simulink model "dft_polyphase_8_channel_builtin_blocks"  (R2018b)
settings: Solver=FixedStepDiscrete  StartTime=0.0  StopTime=t(end)  RelTol=1e-3  EnableMultiTasking=on
InitFcn:
  | M = 8; % Number of channels in the filter bank.
  | N = 8;  % Number of taps in each FIR filter.
  | n_out = 4000; % Number of output samples
  | datatypeselector = 'hdl'; % 'double' 'single' 'hdl' 'dsp'
  | [T,B,U,b,u,t,fs] = generate_inputs(M,N,n_out,datatypeselector);
values from neighbouring files (symbols this model uses):
  B = cast(B,'like',T.fir_filter.coeff)    [generate_inputs.m]
  fs = n    [generate_inputs.m]
libraries: dft_polyphase_channelizer_library x8, dspsrcs4 x1, dspxfrm3 x1
settings Model: Creator=tbryan  LastModifiedBy=tbryan
settings SolverCC: AutoInsertRateTranBlk=on
settings OptimizationCC: LifeSpan=inf
settings DebuggingCC: AllowSymbolicDim=off  SFUnexpectedBacktrackingDiag=warning  SFNoUnconditionalDefaultTransitionDiag=warning  SFExecutionAtInitializationDiag=none
settings SFSimCC: SimUseLocalCustomCode=off
settings RTWCC: RTWUseLocalCustomCode=off
settings CodeAppCC: StateflowObjectComments=on
settings GRTTargetCC: TargetLangStandard=C89/C90 (ANSI)  GeneratePreprocessorConditionals=Disable all
settings ConfigComp: CovMetricSettings=dw  CovHtmlReporting=on  CovSaveCumulativeToWorkspaceVar=on  CovSaveSingleToWorkspaceVar=on  CovExternalEMLEnable=off

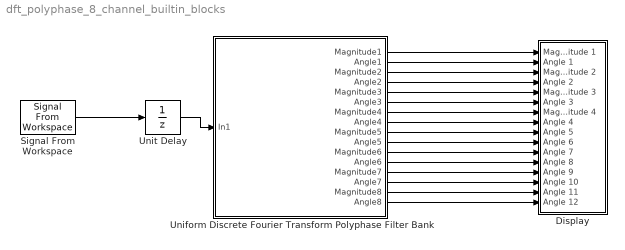
== system dft_polyphase_8_channel_builtin_blocks ==
  Display : Subsystem
  Signal From Workspace : dspsrcs4/Signal From Workspace  X=u  Ts=1/fs  nsamps=1  OutputAfterFinalValue=Setting to zero  ignoreOrWarnInputAndFrameLengths=off  OutputFrames=off
  Uniform Discrete Fourier Transform Polyphase Filter Bank : Subsystem
  Unit Delay : UnitDelay  SampleTime=-1
  wires:
  Signal From Workspace/1 -> Unit Delay/1
  Unit Delay/1 -> Uniform Discrete Fourier Transform Polyphase Filter Bank/1(In1)
  Uniform Discrete Fourier Transform Polyphase Filter Bank/1(Magnitude1) -> Display/1(Magnitude 1)
  Uniform Discrete Fourier Transform Polyphase Filter Bank/2(Angle1) -> Display/2(Angle 1)
  Uniform Discrete Fourier Transform Polyphase Filter Bank/3(Magnitude2) -> Display/3(Magnitude 2)
  Uniform Discrete Fourier Transform Polyphase Filter Bank/4(Angle2) -> Display/4(Angle 2)
  Uniform Discrete Fourier Transform Polyphase Filter Bank/5(Magnitude3) -> Display/5(Magnitude 3)
  Uniform Discrete Fourier Transform Polyphase Filter Bank/6(Angle3) -> Display/6(Angle 3)
  Uniform Discrete Fourier Transform Polyphase Filter Bank/7(Magnitude4) -> Display/7(Magnitude 4)
  Uniform Discrete Fourier Transform Polyphase Filter Bank/8(Angle4) -> Display/8(Angle 4)
  Uniform Discrete Fourier Transform Polyphase Filter Bank/9(Magnitude5) -> Display/9(Angle 5)
  Uniform Discrete Fourier Transform Polyphase Filter Bank/10(Angle5) -> Display/10(Angle 6)
  Uniform Discrete Fourier Transform Polyphase Filter Bank/11(Magnitude6) -> Display/11(Angle 7)
  Uniform Discrete Fourier Transform Polyphase Filter Bank/12(Angle6) -> Display/12(Angle 8)
  Uniform Discrete Fourier Transform Polyphase Filter Bank/13(Magnitude7) -> Display/13(Angle 9)
  Uniform Discrete Fourier Transform Polyphase Filter Bank/14(Angle7) -> Display/14(Angle 10)
  Uniform Discrete Fourier Transform Polyphase Filter Bank/15(Magnitude8) -> Display/15(Angle 11)
  Uniform Discrete Fourier Transform Polyphase Filter Bank/16(Angle8) -> Display/16(Angle 12)

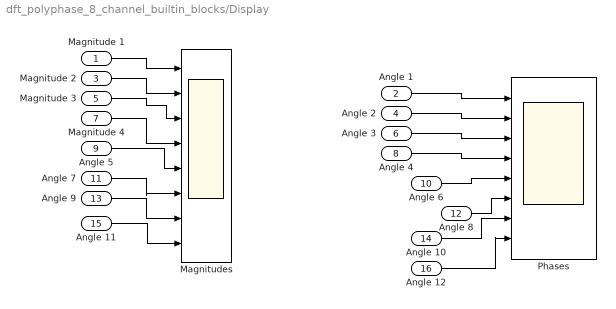
== system dft_polyphase_8_channel_builtin_blocks/Display ==
  Magnitude 1 : Inport
  Angle 1 : Inport  Port=2
  Magnitude 2 : Inport  Port=3
  Angle 2 : Inport  Port=4
  Magnitude 3 : Inport  Port=5
  Angle 3 : Inport  Port=6
  Magnitude 4 : Inport  Port=7
  Angle 4 : Inport  Port=8
  Angle 5 : Inport  Port=9
  Angle 6 : Inport  Port=10
  Angle 7 : Inport  Port=11
  Angle 8 : Inport  Port=12
  Angle 9 : Inport  Port=13
  Angle 10 : Inport  Port=14
  Angle 11 : Inport  Port=15
  Angle 12 : Inport  Port=16
  Magnitudes : Scope  NumInputPorts=8
  Phases : Scope  NumInputPorts=8
  wires:
  Angle 3/1 -> Phases/3
  Magnitude 2/1 -> Magnitudes/2
  Magnitude 1/1 -> Magnitudes/1
  Magnitude 4/1 -> Magnitudes/4
  Angle 2/1 -> Phases/2
  Angle 4/1 -> Phases/4
  Magnitude 3/1 -> Magnitudes/3
  Angle 1/1 -> Phases/1
  Angle 5/1 -> Magnitudes/5
  Angle 7/1 -> Magnitudes/6
  Angle 9/1 -> Magnitudes/7
  Angle 11/1 -> Magnitudes/8
  Angle 6/1 -> Phases/5
  Angle 8/1 -> Phases/6
  Angle 10/1 -> Phases/7
  Angle 12/1 -> Phases/8

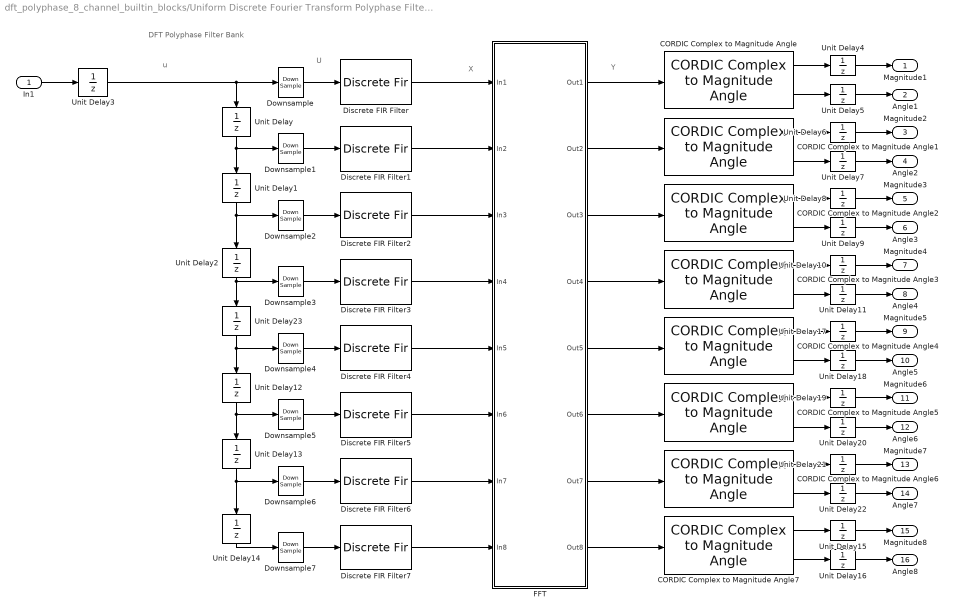
== system dft_polyphase_8_channel_builtin_blocks/Uniform Discrete Fourier Transform Polyphase Filter Bank ==
  note: DFT Polyphase Filter Bank
  note: U
  note: u
  note: X
  note: Y
  In1 : Inport
   CORDIC Complex to Magnitude Angle{,1..7} (8 alike) : dft_polyphase_channelizer_library/CORDIC Complex to Magnitude Angle  SystemSampleTime=-1
  Discrete FIR Filter : DiscreteFir  Coefficients=B(1,:)  AccumDataTypeStr=Inherit: Same as product output
  Discrete FIR Filter1 : DiscreteFir  Coefficients=B(2,:)  AccumDataTypeStr=Inherit: Same as product output
  Discrete FIR Filter2 : DiscreteFir  Coefficients=B(3,:)  AccumDataTypeStr=Inherit: Same as product output
  Discrete FIR Filter3 : DiscreteFir  Coefficients=B(4,:)  AccumDataTypeStr=Inherit: Same as product output
  Discrete FIR Filter4 : DiscreteFir  Coefficients=B(5,:)  AccumDataTypeStr=Inherit: Same as product output
  Discrete FIR Filter5 : DiscreteFir  Coefficients=B(6,:)  AccumDataTypeStr=Inherit: Same as product output
  Discrete FIR Filter6 : DiscreteFir  Coefficients=B(7,:)  AccumDataTypeStr=Inherit: Same as product output
  Discrete FIR Filter7 : DiscreteFir  Coefficients=B(8,:)  AccumDataTypeStr=Inherit: Same as product output
  Downsample{,1..7} (8 alike) : DownSample  N=M  RateOptions=Allow multirate processing
  FFT : Subsystem
      mask Display: disp('IDFT')
  Unit Delay{,1..23} (24 alike) : UnitDelay  SampleTime=-1
  Magnitude1 : Outport
  Angle1 : Outport  Port=2
  Magnitude2 : Outport  Port=3
  Angle2 : Outport  Port=4
  Magnitude3 : Outport  Port=5
  Angle3 : Outport  Port=6
  Magnitude4 : Outport  Port=7
  Angle4 : Outport  Port=8
  Magnitude5 : Outport  Port=9
  Angle5 : Outport  Port=10
  Magnitude6 : Outport  Port=11
  Angle6 : Outport  Port=12
  Magnitude7 : Outport  Port=13
  Angle7 : Outport  Port=14
  Magnitude8 : Outport  Port=15
  Angle8 : Outport  Port=16
  wires:
  FFT/1(Out1) -> " CORDIC Complex to Magnitude Angle"/1
  FFT/2(Out2) -> " CORDIC Complex to Magnitude Angle1"/1
  FFT/3(Out3) -> " CORDIC Complex to Magnitude Angle2"/1
  FFT/4(Out4) -> " CORDIC Complex to Magnitude Angle3"/1
  Unit Delay1/1 -> Unit Delay2/1, Downsample2/1
  Discrete FIR Filter1/1 -> FFT/2(In2)
  Unit Delay/1 -> Unit Delay1/1, Downsample1/1
  Discrete FIR Filter/1 -> FFT/1(In1)
  Discrete FIR Filter2/1 -> FFT/3(In3)
  Discrete FIR Filter3/1 -> FFT/4(In4)
  Downsample3/1 -> Discrete FIR Filter3/1
  Downsample2/1 -> Discrete FIR Filter2/1
  Downsample1/1 -> Discrete FIR Filter1/1
  Downsample/1 -> Discrete FIR Filter/1
  In1/1 -> Unit Delay3/1
  Unit Delay3/1 -> Unit Delay/1, Downsample/1
  Unit Delay4/1 -> Magnitude1/1
  " CORDIC Complex to Magnitude Angle"/1 -> Unit Delay4/1
  Unit Delay5/1 -> Angle1/1
  " CORDIC Complex to Magnitude Angle"/2 -> Unit Delay5/1
  Unit Delay6/1 -> Magnitude2/1
  " CORDIC Complex to Magnitude Angle1"/1 -> Unit Delay6/1
  Unit Delay7/1 -> Angle2/1
  " CORDIC Complex to Magnitude Angle1"/2 -> Unit Delay7/1
  Unit Delay8/1 -> Magnitude3/1
  " CORDIC Complex to Magnitude Angle2"/1 -> Unit Delay8/1
  Unit Delay9/1 -> Angle3/1
  " CORDIC Complex to Magnitude Angle2"/2 -> Unit Delay9/1
  Unit Delay10/1 -> Magnitude4/1
  " CORDIC Complex to Magnitude Angle3"/1 -> Unit Delay10/1
  Unit Delay11/1 -> Angle4/1
  " CORDIC Complex to Magnitude Angle3"/2 -> Unit Delay11/1
  Discrete FIR Filter6/1 -> FFT/7(In7)
  Discrete FIR Filter7/1 -> FFT/8(In8)
  Downsample5/1 -> Discrete FIR Filter5/1
  Discrete FIR Filter4/1 -> FFT/5(In5)
  Unit Delay13/1 -> Unit Delay14/1, Downsample6/1
  Unit Delay12/1 -> Unit Delay13/1, Downsample5/1
  Downsample4/1 -> Discrete FIR Filter4/1
  Downsample6/1 -> Discrete FIR Filter6/1
  Discrete FIR Filter5/1 -> FFT/6(In6)
  Downsample7/1 -> Discrete FIR Filter7/1
  Unit Delay14/1 -> Downsample7/1
  Unit Delay2/1 -> Unit Delay23/1, Downsample3/1
  Unit Delay21/1 -> Magnitude7/1
  Unit Delay15/1 -> Magnitude8/1
  " CORDIC Complex to Magnitude Angle6"/1 -> Unit Delay21/1
  Unit Delay16/1 -> Angle8/1
  " CORDIC Complex to Magnitude Angle7"/1 -> Unit Delay15/1
  " CORDIC Complex to Magnitude Angle5"/2 -> Unit Delay20/1
  Unit Delay22/1 -> Angle7/1
  " CORDIC Complex to Magnitude Angle4"/1 -> Unit Delay17/1
  " CORDIC Complex to Magnitude Angle7"/2 -> Unit Delay16/1
  Unit Delay17/1 -> Magnitude5/1
  Unit Delay19/1 -> Magnitude6/1
  " CORDIC Complex to Magnitude Angle6"/2 -> Unit Delay22/1
  " CORDIC Complex to Magnitude Angle5"/1 -> Unit Delay19/1
  Unit Delay20/1 -> Angle6/1
  Unit Delay18/1 -> Angle5/1
  " CORDIC Complex to Magnitude Angle4"/2 -> Unit Delay18/1
  FFT/5(Out5) -> " CORDIC Complex to Magnitude Angle4"/1
  FFT/6(Out6) -> " CORDIC Complex to Magnitude Angle5"/1
  FFT/7(Out7) -> " CORDIC Complex to Magnitude Angle6"/1
  FFT/8(Out8) -> " CORDIC Complex to Magnitude Angle7"/1
  Unit Delay23/1 -> Unit Delay12/1, Downsample4/1

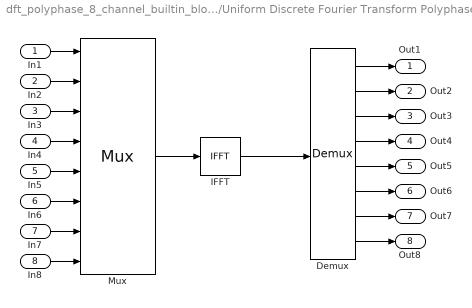
== system dft_polyphase_8_channel_builtin_blocks/Uniform Discrete Fourier Transform Polyphase Filter Bank/FFT ==
  In1 : Inport
  In2 : Inport  Port=2
  In3 : Inport  Port=3
  In4 : Inport  Port=4
  In5 : Inport  Port=5
  In6 : Inport  Port=6
  In7 : Inport  Port=7
  In8 : Inport  Port=8
  Demux : Demux  Outputs=8
  IFFT : dspxfrm3/IFFT  FFTImplementation=Auto  CompMethod=Table lookup  TableOpt=NEW  TableOptActive=Speed  BitRevOrder=off  cs_in=off  Normalize=on  InheritFFTLength=on  FFTLength=64  WrapInput=on  mode=Complex  outSamplingMode=Sample based  roundingMode=Floor  overflowMode=off  firstCoeffDataTypeStr=Inherit: Same word length as input  firstCoeffLastDataTypeStr=Inherit: Same word length as input  outputMin=[]  outputMax=[]
      settings: SourceProductName=DSP System Toolbox
  Mux : Mux  Inputs=8
  Out1 : Outport
  Out2 : Outport  Port=2
  Out3 : Outport  Port=3
  Out4 : Outport  Port=4
  Out5 : Outport  Port=5
  Out6 : Outport  Port=6
  Out7 : Outport  Port=7
  Out8 : Outport  Port=8
  wires:
  Mux/1 -> IFFT/1
  IFFT/1 -> Demux/1
  In1/1 -> Mux/1
  In4/1 -> Mux/4
  In3/1 -> Mux/3
  In2/1 -> Mux/2
  Demux/2 -> Out2/1
  Demux/3 -> Out3/1
  Demux/4 -> Out4/1
  Demux/1 -> Out1/1
  In5/1 -> Mux/5
  In6/1 -> Mux/6
  In7/1 -> Mux/7
  In8/1 -> Mux/8
  Demux/5 -> Out5/1
  Demux/8 -> Out8/1
  Demux/7 -> Out7/1
  Demux/6 -> Out6/1
